simulink model "lab11"  (R2016b)
settings: Solver=FixedStepAuto  StartTime=0.0  StopTime=0.006  FixedStep=6e-8  RelTol=1e-3  EnableMultiTasking=on
settings Model: Creator=Niirn  LastModifiedBy=Niirn
settings DataIOCC: LimitDataPoints=on  SaveFormat=Array
settings OptimizationCC: LifeSpan=inf
settings DebuggingCC: UnderspecifiedInitializationDetection=Classic  MergeDetectMultiDrivingBlocksExec=none  SolverPrmCheckMsg=warning  SFUnexpectedBacktrackingDiag=warning  SFNoUnconditionalDefaultTransitionDiag=warning  SFExecutionAtInitializationDiag=none
settings HardwareCC: ProdBitPerPointer=32  ProdBitPerSizeT=32  ProdBitPerPtrDiffT=32  ProdLargestAtomicFloat=None  ProdIntDivRoundTo=Undefined  ProdEndianess=Unspecified  ProdWordSize=32  ProdHWDeviceType=32-bit Generic
settings ModelReferenceCC: PropagateSignalLabelsOutOfModel=off
settings GRTTargetCC: TargetLangStandard=C89/C90 (ANSI)  GeneratePreprocessorConditionals=Disable all
settings ConfigComp: CovMetricSettings=dw  CovHtmlReporting=on  CovSaveCumulativeToWorkspaceVar=on  CovSaveSingleToWorkspaceVar=on  CovExternalEMLEnable=off

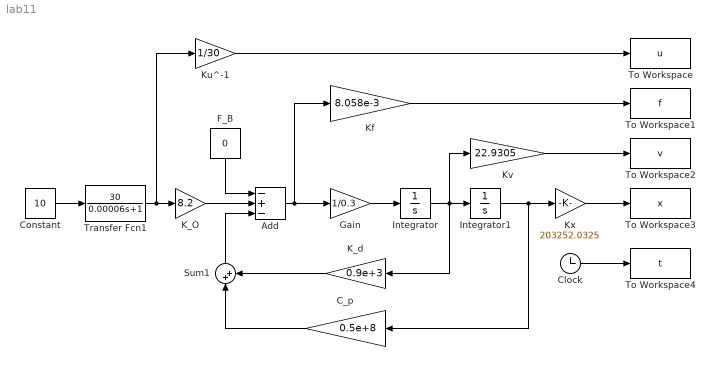
== system lab11 ==
  Add : Sum  Inputs=-+-
  C_p : Gain  Gain=0.5e+8
  Clock : Clock
  Constant : Constant  Value=10
  F_B : Constant  Value=0
  Gain : Gain  Gain=1/0.3
  Integrator : Integrator
  Integrator1 : Integrator
  K_O : Gain  Gain=8.2
  K_d : Gain  Gain=0.9e+3
  Kf : Gain  Gain=8.058e-3
  Ku^-1 : Gain  Gain=1/30
  Kv : Gain  Gain=22.9305
  Kx : Gain  Gain=203252.0325
  Sum1 : Sum  Inputs=|++
  To Workspace : ToWorkspace  VariableName=u  SampleTime=-1
  To Workspace1 : ToWorkspace  VariableName=f  SampleTime=-1
  To Workspace2 : ToWorkspace  VariableName=v  SampleTime=-1
  To Workspace3 : ToWorkspace  VariableName=x  SampleTime=-1
  To Workspace4 : ToWorkspace  VariableName=t  SampleTime=-1
  Transfer Fcn1 : TransferFcn  Numerator=[30]  Denominator=[0.00006 1]
  wires:
  Gain/1 -> Integrator/1
  Integrator/1 -> Kv/1, K_d/1, Integrator1/1
  Integrator1/1 -> Kx/1, C_p/1
  K_d/1 -> Sum1/2
  C_p/1 -> Sum1/1
  Constant/1 -> Transfer Fcn1/1
  Transfer Fcn1/1 -> Ku^-1/1, K_O/1
  Add/1 -> Gain/1, Kf/1
  Sum1/1 -> Add/3
  K_O/1 -> Add/2
  F_B/1 -> Add/1
  Kx/1 -> To Workspace3/1
  Kv/1 -> To Workspace2/1
  Kf/1 -> To Workspace1/1
  Ku^-1/1 -> To Workspace/1
  Clock/1 -> To Workspace4/1
